simulink model "EV_thermal_charger_2015a_jmaab_Can02"  (R2015a)
settings: Solver=ode3  StartTime=0.0  StopTime=1800  FixedStep=sampling_time  RelTol=1e-3
PreLoadFcn:
  | %run('init_setting.m')
PostLoadFcn:
  | %set_param(gcs, 'SimulationCommand', 'update');
  | %load('save_param/save_P_Charger', 'P_Charger');
  | %load('save_param/save_T_User_set_temp_degC','T_User_set_temp_degC');
  | %load('save_param/save_ENV_PNT_PTTH_Temp_add_degC','ENV_PNT_PTTH_Temp_add_degC');
  | %load('save_param/save_ENV_PNT_CABIN_Temp_add_degC','ENV_PNT_CABIN_Temp_add_degC');
  | %load('save_param/save_ENV_PNT_PHI_Sunlight_W','ENV_PNT_PHI_Sunlight_W');
  | %load('save_param/save_ENV_PNT_Outside_Temp_ini_degC','ENV_PNT_Outside_Temp_ini_degC');
StartFcn:
  | tic
StopFcn:
  | toc
  | disp(['実時間の' num2str(toc/max(tout)) '倍'])
undefined symbols (not defined in the file or in its folder): BK_PNT_Pow_UL, BK_PNT_ReGene_vel_limit_DN_kmph, BK_PNT_ReGene_vel_limit_UP_kmph, BK_PNT_Tau_brake, Brk_LL, Brk_PGain, Brk_UL, BT_PNT_Hi_C_pol_hi_batt, BT_PNT_Hi_Capa_hi_batt_F, BT_PNT_Hi_ocv_SOC_hi_batt_OCV_V_table, BT_PNT_Hi_ocv_SOC_hi_batt_OCV_V_table_x_SOC, BT_PNT_Hi_R_hi_batt_cell, BT_PNT_Hi_R_pol_hi_batt, BT_PNT_Hi_SOC_MAX_hi_batt, BT_PNT_Hi_SOC_MIN_hi_batt, BT_PNT_Hi_SOC_START_hi_batt, BT_PNT_Lo_Capa_lo_batt_F, BT_PNT_Lo_ocv_SOC_lo_batt_OCV_V_table, BT_PNT_Lo_ocv_SOC_lo_batt_OCV_V_table_x_SOC, BT_PNT_Lo_R_lo_batt_ohm, BT_PNT_Lo_SOC_MAX_lo_batt, BT_PNT_Lo_SOC_MIN_lo_batt, BT_PNT_Lo_SOC_START_lo_batt, BTTH_CNT_P_BT_Heater_W, BTTH_CNT_P_BT_Heater_W_x_BTCells_degC, BTTH_CNT_Voltage_BTFan_V, BTTH_CNT_Voltage_BTFan_V_x_BTCells_degC, BTTH_PNT_BT_Heat_Resi_KpW, BTTH_PNT_BT_Heat_Resi_KpW_x_Wind_m3ps, BTTH_PNT_BT_Heater2BTCells_Heat_Resi_KpW, BTTH_PNT_BT_Heater_Heat_Capa_JpK, BTTH_PNT_BTBlock2BTAir_Heat_Resi_KpW, BTTH_PNT_BTBlock_Heat_Capa_JpK, BTTH_PNT_BTCells2BTBlock_Heat_Resi_KpW, BTTH_PNT_BTCells_Heat_Capa_JpK, BTTH_PNT_v_BTFan_Wind_vel_mps, BTTH_PNT_v_BTFan_Wind_vel_mps_x_V_BTFan, CATH_CNT_P_Aircon_W_LL, CATH_CNT_P_Aircon_W_UL, CATH_CNT_P_Gain_Aircon, CATH_CNT_P_Gain_PTC_Heater, CATH_CNT_P_Gain_SeatHT, CATH_CNT_P_PTC_Heater, CATH_CNT_P_PTC_Heater_W_LL, CATH_CNT_P_PTC_Heater_W_UL, CATH_CNT_P_PTC_Heater_x_T_Outside_temp_degC, CATH_CNT_P_SeatHT_W_LL, CATH_CNT_P_SeatHT_W_UL, CATH_CNT_PGain_Temp_blowout, CATH_CNT_T_Aircon_Indoor_degC, CATH_CNT_T_Aircon_Indoor_degC_x_T_blowout_degC, CATH_CNT_T_PTC_Heater_degC_UL, CATH_CNT_T_SeatHT_Temp_degC, CATH_CNT_T_SeatHT_Temp_degC_x_T_blowout_degC, CATH_CNT_V_HVAC_Fan, CATH_CNT_V_HVAC_Fan_x_T_blowout_degC, CATH_CNT_V_RDFan_V, CATH_CNT_V_RDFan_x_P_Aircon_W, CATH_PNT_Air_Convection_Heat_Resi_KpW, CATH_PNT_Air_Convection_Heat_Resi_x_mps ... (+141)
undefined symbols (not defined in the file): ACC_D_Gain, ACC_I_Gain, ACC_P_Gain
libraries: METI_Lib_vehicle_model x52, simulink x35
(part 2 of 6)

== system EV_thermal_charger_2015a_jmaab_Can02/Vehicle/EL_PNT ==
  note: 抵抗性負荷
  V_BT_Lo_PNT_V : Inport
  Add : Sum  Inputs=-+|
  Constant : Constant  Value=EL_PNT_R_bodyelec_lo
  Divide_0wari1 : Subsystem  mask(Divide_0割防止){}
      mask help:
      | 0割防止を行ったDivideブロックです。
      | 第2入力端子が0の場合、出力は0になります。
      mask Help:
      | 0割防止を行ったDivideブロックです。
      | 第2入力端子が0の場合、出力は0になります。
      mask Display:
      | port_label('input', 1, '×')
      | port_label('input', 2, '÷')
  Gain : Gain  Gain=-1
  Lo_body_elec_load_resi : Subsystem
  P_cal : METI_Lib_vehicle_model/P_cal  Type_energy=電気  Type_output_energy=損失  Power_name=Pl_  t_Workspace_Name=EL_PNT  P_VariableName=Pl_EL_PNT  Across_VariableName=V_EL_PNT  Throgh_VariableName=I_EL_PNT
  Terminator1 : Terminator
  V_Body_ground : Constant  Value=0
  I_EL_PNT_A : Outport
  wires:
  Divide_0wari1/1(Out1) -> Gain/1, P_cal/2
  V_BT_Lo_PNT_V/1 -> Add/2, P_cal/1
  Gain/1 -> I_EL_PNT_A/1  "I_EL_PNT_A"
  P_cal/1 -> Terminator1/1
  Constant/1 -> Divide_0wari1/2(In2)
  Add/1 -> Divide_0wari1/1(In1)
  V_Body_ground/1 -> Add/1

== system EV_thermal_charger_2015a_jmaab_Can02/Vehicle/INV_PT ==
  MG_CNT_out : Inport
  V_BT_Hi_PNT_V : Inport  Port=2
  T_INVTH_PNT_K : Inport  Port=3
  V_MG_PNT_AC_V : Inport  Port=4
  Bus Creator3 : BusCreator
  Bus Creator4 : BusCreator  Inputs=2
  Bus Selector8 : BusSelector  OutputSignals=tgt_I_MG_CNT_UPhase_A,tgt_k_MG_CNT_Vpradps,Power_factor_MG_CNT
  INV_PNT : Subsystem
  INV_sensor : Outport
  INV_MG : Outport  Port=2
  I_INV_PNT_AC_A : Outport  Port=3
  PHI_INV_PNT_W : Outport  Port=4
  I_INV_PNT_DC_A : Outport  Port=5
  wires:
  INV_PNT/2(Power_factor_INV_PNT) -> Bus Creator3/2, Bus Creator4/1  "Power_factor_INV_PNT"
  INV_PNT/3(V_INV_PNT_DC_V) -> Bus Creator3/3  "V_INV_PNT_DC_V"
  INV_PNT/1(k_INV_PNT_Vpradps) -> Bus Creator4/2, Bus Creator3/1  "k_INV_PNT_Vpradps"
  Bus Selector8/3 -> INV_PNT/3(Power_factor_MG_CNT)  "<Power_factor_MG_CNT>"
  T_INVTH_PNT_K/1 -> INV_PNT/5(T_INVTH_PNT_K)
  INV_PNT/4(I_INV_PNT_DC_A_1) -> Bus Creator3/4  "I_INV_PNT_DC_A_1"
  Bus Selector8/2 -> INV_PNT/2(tgt_k_MG_CNT_vpradps)  "<tgt_k_MG_CNT_Vpradps>"
  Bus Selector8/1 -> INV_PNT/1(tgt_I_MG_CNT_UPhase_A)  "<tgt_I_MG_CNT_UPhase_A>"
  V_BT_Hi_PNT_V/1 -> INV_PNT/4(V_BT_Hi_PNT_V)
  INV_PNT/5(I_INV_PNT_AC_A) -> I_INV_PNT_AC_A/1
  INV_PNT/7(I_INV_PNT_DC_A) -> I_INV_PNT_DC_A/1
  INV_PNT/6(PHI_INV_PNT_W) -> PHI_INV_PNT_W/1
  V_MG_PNT_AC_V/1 -> INV_PNT/6(V_MG_PNT_AC_V)
  Bus Creator3/1 -> INV_sensor/1  "INV_sensor"
  Bus Creator4/1 -> INV_MG/1  "INV_MG"
  MG_CNT_out/1 -> Bus Selector8/1

== system EV_thermal_charger_2015a_jmaab_Can02/Vehicle/MG_PNT ==
  INV_MG : Inport
  I_INV_PNT_AC_A : Inport  Port=2
  T_MGTH_PNT_K : Inport  Port=3
  w_TM_PNT_UP_radps : Inport  Port=4
  Bus Creator2 : BusCreator
  Bus Selector5 : BusSelector  OutputSignals=k_INV_PNT_Vpradps,Power_factor_INV_PNT
  MG_PNT : Subsystem
  MG_sensor : Outport
  Trq_MG_PNT_Nm : Outport  Port=2
  V_MG_PNT_AC_V : Outport  Port=3
  PHI_MG_PNT_W : Outport  Port=4
  wires:
  MG_PNT/3(V_MG_PNT_AC_V_1) -> Bus Creator2/3  "V_MG_PNT_AC_V_1"
  Bus Selector5/1 -> MG_PNT/1(k_MG_CNT_Vpradps)  "<k_INV_PNT_Vpradps>"
  T_MGTH_PNT_K/1 -> MG_PNT/4(T_MGTH_PNT_K)
  MG_PNT/1(w_MG_PNT_radps) -> Bus Creator2/1  "w_MG_PNT_radps"
  Bus Selector5/2 -> MG_PNT/2(Power_factor_INV_PNT)  "<Power_factor_INV_PNT>"
  MG_PNT/2("Trq_MG_PNT_Nm_1 ") -> Bus Creator2/2  "Trq_MG_PNT_Nm_1"
  MG_PNT/6("PHI_MG_PNT_W ") -> PHI_MG_PNT_W/1
  INV_MG/1 -> Bus Selector5/1
  MG_PNT/4(I_MG_PNT_AC_A) -> Bus Creator2/4  "I_MG_PNT_AC_A"
  Bus Creator2/1 -> MG_sensor/1  "MG_sensor"
  I_INV_PNT_AC_A/1 -> MG_PNT/3("I_INV_PNT_AC_A ")
  MG_PNT/5(Trq_MG_PNT_Nm) -> Trq_MG_PNT_Nm/1
  w_TM_PNT_UP_radps/1 -> MG_PNT/5(w_TM_PNT_UP_radps)
  MG_PNT/7("V_MG_PNT_AC_V ") -> V_MG_PNT_AC_V/1

== system EV_thermal_charger_2015a_jmaab_Can02/Vehicle/TR_PNT ==
  note: 車両を動かす側が正
  note: 車両を動かす側が正
  note: M (トルクNm) = F (力(N)） × r (タイヤ半径(m))
  note: omg (回転数rad/s) = v (車速m/s) / r (タイヤ半径(m))
  note: トルク⇔力変換
  note: 並進⇔回転変換
  note: 転がり抵抗
  "Trq_TR_PNT_Nm " : Inport
  Trq_TR_PNT_Nm 1 : Inport  Port=2
  v_VL_PNT_mps : Inport  Port=3
  Add5 : Sum
  Constant2 : Constant  Value=1/tire_r
  Product5 : Product  RndMeth=Zero
  Product6 : Product  RndMeth=Zero
  Sum2 : Sum  Inputs=-+|
  cal_roll_resi : METI_Lib_vehicle_model/vehicle_model/cal_roll_resi  Myu_tire=myu  Vehicle_Mass=M  Gravi_acc=g
  "F_TR_PNT_N " : Outport
  ｗ_TR_PNT_radps : Outport  Port=2
  tag scope: tScope_F_tire=global
  wires:
  "Trq_TR_PNT_Nm "/1 -> Add5/1
  Product5/1 -> ｗ_TR_PNT_radps/1  "w_TR_PNT_radps"
  v_VL_PNT_mps/1 -> Product5/1, cal_roll_resi/1
  Constant2/1 -> Product6/1, Product5/2
  Product6/1 -> Sum2/2
  cal_roll_resi/1 -> Sum2/1
  Sum2/1 -> "F_TR_PNT_N "/1, [tScope_F_tire]  "f_TR_PNT_N"
  Add5/1 -> Product6/2
  Trq_TR_PNT_Nm 1/1 -> Add5/2

== system EV_thermal_charger_2015a_jmaab_Can02/Vehicle/VL_PNT ==
  note: 空気抵抗
  note: 登坂抵抗
  note: 車両慣性
  F_TR_PNT_N : Inport
  Bus Creator : BusCreator  Inputs=1
  P_cal : METI_Lib_vehicle_model/P_cal  Type_energy=並進運動  Type_output_energy=出力  Power_name=Po_  t_Workspace_Name=VL_PNT_TIRE_MECK  P_VariableName=Po_VL_PNT_TIRE_MECK  Across_VariableName=v_VL_PNT_TIRE_MECK  Throgh_VariableName=F_VL_PNT_TIRE_MECK
  P_cal1 : METI_Lib_vehicle_model/P_cal  Type_energy=並進運動  Type_output_energy=損失  Power_name=Pl_  t_Workspace_Name=VL_PNT_AIR_RESI  P_VariableName=Pl_VL_PNT_AIR_RESI  Across_VariableName=v_VL_PNT_AIR_RESI  Throgh_VariableName=F_VL_PNT_AIR_RESI
  P_cal3 : METI_Lib_vehicle_model/P_cal  Type_energy=並進運動  Type_output_energy=損失  Power_name=Pl_  t_Workspace_Name=VL_PNT_GRAD_RESI_MECK  P_VariableName=Pl_VL_PNT_GRAD_RESI_MECK  Across_VariableName=v_VL_PNT_GRAD_RESI_MECK  Throgh_VariableName=F_VL_PNT_GRAD_RESI_MECK
  P_cal4 : METI_Lib_vehicle_model/P_cal  Type_energy=並進運動  Type_output_energy=出力  Power_name=Po_  t_Workspace_Name=VL_PNT_VL_MASS_MECK  P_VariableName=Po_VL_PNT_VL_MASS_MECK  Across_VariableName=v_VL_PNT_VL_MASS_MECK  Throgh_VariableName=F_VL_PNT_VL_MASS_MECK
  Sum1 : Sum  Inputs=-+|
  Sum3 : Sum  Inputs=-+|
  Terminator{2..5} (4 alike) : Terminator
  V_wind : Constant  Value=0
  angle : Constant  Value=0
  cal_Air_resi : METI_Lib_vehicle_model/vehicle_model/cal_Air_resi  Vel_max=200
  cal_Hill_Climbing_Resi : Subsystem
      mask Display: image(imread('picture\登坂.JPG'))
  cal_Vehicle_Mass : METI_Lib_vehicle_model/vehicle_model/cal_Vehicle_Mass  Vehicle_Mass=M
  mps2kmph : Gain  Gain=mps2kmph
  VL_PNT_sensor : Outport
  v_VL_PNT_mps : Outport  Port=2
  wires:
  P_cal4/1 -> Terminator2/1
  Sum1/1 -> cal_Vehicle_Mass/1, P_cal4/2
  P_cal1/1 -> Terminator5/1
  V_wind/1 -> cal_Air_resi/2
  cal_Air_resi/1 -> P_cal1/2, Sum3/1
  F_TR_PNT_N/1 -> P_cal/2, Sum3/2
  P_cal/1 -> Terminator3/1
  cal_Hill_Climbing_Resi/1(Out1) -> P_cal3/2, Sum1/1
  P_cal3/1 -> Terminator4/1
  Sum3/1 -> Sum1/2
  angle/1 -> cal_Hill_Climbing_Resi/1(In1)
  cal_Vehicle_Mass/1 -> mps2kmph/1, P_cal4/1, v_VL_PNT_mps/1, P_cal3/1, P_cal/1, P_cal1/1, cal_Air_resi/1  "v_VL_PNT_mps"
  mps2kmph/1 -> Bus Creator/1  "v_VL_PNT_kmph"
  Bus Creator/1 -> VL_PNT_sensor/1  "VL_PNT_sensor"

== system EV_thermal_charger_2015a_jmaab_Can02/Driver/Caliculate_Opeining_Accel/FB ==
  delta_v_VL_kmph : Inport
  Acc_D_Gain : Gain  Gain=D_Gain
  Acc_I_Gain : Gain  Gain=I_Gain
  Acc_P_Gain : Gain  Gain=P_Gain
  Acc_P_Gain1 : Gain  Gain=P_Gain
  Derivative : Derivative
  Filter : Subsystem  Commented=through
  Integrator : Integrator
  Memory : Memory
  Product1 : Product
  Saturation2 : Saturate  UpperLimit=1  LowerLimit=0
  Sum : Sum  Inputs=+++
  Terminator : Terminator
  FB_open_accel_per : Outport
  wires:
  Filter/1(Out1) -> Product1/2
  Saturation2/1 -> Acc_P_Gain/1
  Acc_P_Gain/1 -> Product1/1
  Sum/1 -> FB_open_accel_per/1
  Derivative/1 -> Acc_D_Gain/1
  Integrator/1 -> Acc_I_Gain/1
  delta_v_VL_kmph/1 -> Memory/1
  Acc_I_Gain/1 -> Sum/3
  Acc_D_Gain/1 -> Sum/2
  Acc_P_Gain1/1 -> Sum/1
  Memory/1 -> Saturation2/1, Filter/1(In1), Acc_P_Gain1/1, Integrator/1, Derivative/1
  Product1/1 -> Terminator/1

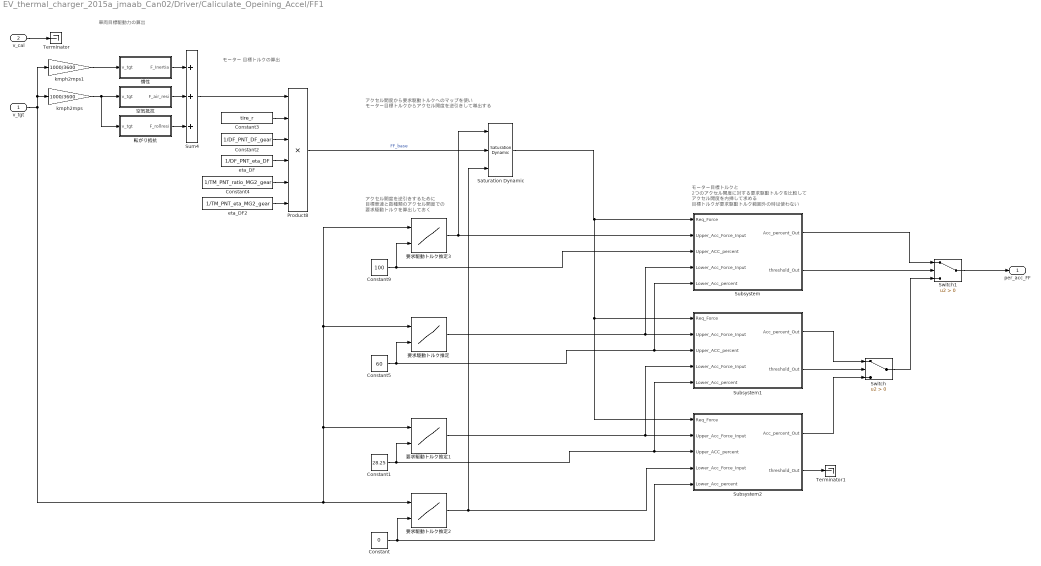
== system EV_thermal_charger_2015a_jmaab_Can02/Driver/Caliculate_Opeining_Accel/FF1 ==
  note: モーター目標トルクと
      | 2つのアクセル開度に対する要求駆動トルクを比較して
      | アクセル開度を内挿して求める
      | 目標トルクが要求駆動トルク範囲外の時は使わない
  note: アクセル開度を逆引きするために
      | 目標車速と数種類のアクセル開度での
      | 要求駆動トルクを算出しておく
  note: アクセル開度から要求駆動トルクへのマップを使い
      | モーター目標トルクからアクセル開度を逆引きして導出する
  note: モーター 目標トルクの算出
  note: 車両目標駆動力の算出
  v_tgt : Inport
  v_cal : Inport  Port=2
  Constant : Constant  Value=0
  Constant1 : Constant  Value=28.25
  Constant2 : Constant  Value=1/DF_PNT_DF_gear
  Constant3 : Constant  Value=tire_r
  Constant4 : Constant  Value=1/TM_PNT_ratio_MG2_gear
  Constant5 : Constant  Value=60
  Constant9 : Constant  Value=100
  Product8 : Product  Inputs=******  RndMeth=Zero
  Saturation Dynamic : simulink/Discontinuities/Saturation Dynamic  OutMin=[]  OutMax=[]  OutDataTypeStr=Inherit: Same as second input  OutDataType=fixdt(1, 16)  OutScaling=2^-10  DoSatur=off
  Subsystem : Subsystem
  Subsystem1 : Subsystem
  Subsystem2 : Subsystem
  Sum4 : Sum  Inputs=+++
  Switch : Switch  Criteria=u2 > Threshold
  Switch1 : Switch  Criteria=u2 > Threshold
  Terminator : Terminator
  Terminator1 : Terminator
  eta_DF : Constant  Value=1/DF_PNT_eta_DF
  eta_DF2 : Constant  Value=1/TM_PNT_eta_MG2_gear
  kmph2mps : Gain  Gain=1000/3600
  kmph2mps1 : Gain  Gain=1000/3600
  慣性 : Subsystem
  空気抵抗 : Subsystem
  要求駆動トルク推定{,1..3} (4 alike) : Lookup_n-D  BreakpointsForDimension1=VCU_CNT_trq_require_v_kmph  BreakpointsForDimension2=VCU_CNT_trq_require_accper  BeginIndexSearchUsingPreviousIndexResult=on  Table=VCU_CNT_trq_require_Nm  ExtrapMethod=Clip  InternalRulePriority=Speed  RndMeth=Simplest  InputSameDT=on
  転がり抵抗 : Subsystem
  per_acc_FF : Outport
  wires:
  v_cal/1 -> Terminator/1
  kmph2mps/1 -> 空気抵抗/1(v_tgt), 転がり抵抗/1(v_tgt)
  kmph2mps1/1 -> 慣性/1(v_tgt)
  慣性/1(F_Inertia) -> Sum4/1
  転がり抵抗/1(F_rollresi) -> Sum4/3
  空気抵抗/1(F_air_resi) -> Sum4/2
  Sum4/1 -> Product8/1
  v_tgt/1 -> kmph2mps/1, kmph2mps1/1, 要求駆動トルク推定2/1, 要求駆動トルク推定1/1, 要求駆動トルク推定3/1, 要求駆動トルク推定/1
  Constant/1 -> 要求駆動トルク推定2/2, Subsystem2/5(Lower_Acc_percent)
  Constant1/1 -> 要求駆動トルク推定1/2, Subsystem2/3(Upper_ACC_percent), Subsystem1/5(Lower_Acc_percent)
  Constant5/1 -> 要求駆動トルク推定/2, Subsystem1/3(Upper_ACC_percent), Subsystem/5(Lower_Acc_percent)
  要求駆動トルク推定1/1 -> Subsystem1/4(Lower_Acc_Force_Input), Subsystem2/2(Upper_Acc_Force_Input)
  要求駆動トルク推定2/1 -> Saturation Dynamic/3, Subsystem2/4(Lower_Acc_Force_Input)
  Product8/1 -> Saturation Dynamic/2  "FF_base"
  Saturation Dynamic/1 -> Subsystem1/1(Req_Force), Subsystem2/1(Req_Force), Subsystem/1(Req_Force)
  Constant9/1 -> 要求駆動トルク推定3/2, Subsystem/3(Upper_ACC_percent)
  要求駆動トルク推定/1 -> Subsystem1/2(Upper_Acc_Force_Input), Subsystem/4(Lower_Acc_Force_Input)
  要求駆動トルク推定3/1 -> Subsystem/2(Upper_Acc_Force_Input), Saturation Dynamic/1
  Switch/1 -> Switch1/3
  Switch1/1 -> per_acc_FF/1
  Subsystem/1(Acc_percent_Out) -> Switch1/1
  Subsystem/2(threshold_Out) -> Switch1/2
  Subsystem1/2(threshold_Out) -> Switch/2
  Subsystem1/1(Acc_percent_Out) -> Switch/1
  Subsystem2/1(Acc_percent_Out) -> Switch/3
  Subsystem2/2(threshold_Out) -> Terminator1/1
  Constant3/1 -> Product8/2
  Constant2/1 -> Product8/3
  eta_DF/1 -> Product8/4
  Constant4/1 -> Product8/5
  eta_DF2/1 -> Product8/6

== system EV_thermal_charger_2015a_jmaab_Can02/Driver/Caliculate_Opeining_Accel/stopmode_calc ==
  note: 停車時（＝目標車速が閾値以下の時）は
      | アクセルを踏まないようにする
  FF_FB_acc_per : Inport
  target_v_VL_kmph : Inport  Port=2
  Compare To Zero : simulink/Logic and Bit Operations/Compare To Zero  relop=>  OutDataTypeStr=boolean
  Constant2 : Constant  Value=0
  Constant6 : Constant  Value=Driver_Brake_Switch_Const2
  Subtract : Sum  Inputs=+-
  Switch : Switch  Criteria=u2 > Threshold
  open_accel_per : Outport
  wires:
  Subtract/1 -> Compare To Zero/1
  Switch/1 -> open_accel_per/1
  Compare To Zero/1 -> Switch/2
  Constant2/1 -> Switch/3
  Constant6/1 -> Subtract/2
  target_v_VL_kmph/1 -> Subtract/1
  FF_FB_acc_per/1 -> Switch/1

== system EV_thermal_charger_2015a_jmaab_Can02/Vehicle/ATM_PNT/degC->K ==
  degC : Inport
  Constant2 : Constant  Value=degC2K
  Sum : Sum  Inputs=++|
  K : Outport
  wires:
  degC/1 -> Sum/2
  Constant2/1 -> Sum/1
  Sum/1 -> K/1

== system EV_thermal_charger_2015a_jmaab_Can02/Vehicle/BAT_Hi_PNT/BT_Hi_PNT ==
  note: SOC算出
  note: 内部抵抗
  note: OCV電圧算出
  I_BT_Hi_PNT_A : Inport
  T_BC_PNT_K : Inport  Port=2
  Cal_SOC : Subsystem
  Capa_batt(Ah) : Constant  Value=BT_PNT_Hi_Capa_hi_batt_F
  Gain : Gain  Gain=-1
  Memory6 : Memory  InheritSampleTime=on
  P_cal : METI_Lib_vehicle_model/P_cal  Type_energy=電気  Type_output_energy=出力  Power_name=Po_  t_Workspace_Name=BT_HI_PNT_ELEC  P_VariableName=Po_BT_HI_PNT_ELEC  Across_VariableName=V_BT_HI_PNT_ELEC  Throgh_VariableName=I_BT_HI_PNT_ELEC
  P_cal1 : METI_Lib_vehicle_model/P_cal  Type_energy=電気  Type_output_energy=損失  Power_name=Pl_  t_Workspace_Name=BT_PNT_HI_ELEC_LOSS  P_VariableName=Pl_BT_PNT_HI_ELEC_LOSS  Across_VariableName=V_BT_PNT_HI_ELEC_LOSS  Throgh_VariableName=I_BT_PNT_HI_ELEC_LOSS
  Product : Product
  SOC_MAX(%) : Constant  Value=BT_PNT_Hi_SOC_MAX_hi_batt
  SOC_MIN(%) : Constant  Value=BT_PNT_Hi_SOC_MIN_hi_batt
  SOC_START(%) : Constant  Value=BT_PNT_Hi_SOC_START_hi_batt
  Signal Specification : SignalSpecification
  Subsystem : Subsystem
  Sum : Sum
  Terminator1 : Terminator
  Terminator2 : Terminator
  map_OCV : Lookup  InputValues=BT_PNT_Hi_ocv_SOC_hi_batt_OCV_V_table_x_SOC  Table=BT_PNT_Hi_ocv_SOC_hi_batt_OCV_V_table  LookUpMeth=Interpolation-Use End Values
  V_BT_Hi_PNT_V_1 : Outport
  SOC_BT_Hi_PNT_per : Outport  Port=2
  V_BT_Hi_PNT_V : Outport  Port=3
  PHI_BT_Hi_PNT_W : Outport  Port=4
  tag scope: tScope_I_BT_HI_PNT_A=global, tScope_PHI_BT_HI_PNT_W=global, tScope_P_BT_HI_PNT_W=global, tScope_SOC_HiBatt=global, tScope_V_BT_HI_PNT_V=global
  wires:
  Capa_batt(Ah)/1 -> Cal_SOC/2(Capa_batt)
  SOC_START(%)/1 -> Cal_SOC/3(SOC_st)
  SOC_MAX(%)/1 -> Cal_SOC/4(SOC_MAX)
  SOC_MIN(%)/1 -> Cal_SOC/5(SOC_MIN)
  Sum/1 -> V_BT_Hi_PNT_V_1/1, Product/1, Signal Specification/1, [tScope_V_BT_HI_PNT_V], P_cal/1  "volt_BT_HI_PNT_V"
  map_OCV/1 -> Sum/1
  Subsystem/1(V_BT_PNT_V) -> P_cal1/1, Sum/2
  P_cal/1 -> Terminator2/1
  P_cal1/1 -> PHI_BT_Hi_PNT_W/1, [tScope_PHI_BT_HI_PNT_W]  "PHI_BT_Hi_PNT_W"
  I_BT_Hi_PNT_A/1 -> Gain/1, Memory6/1
  Cal_SOC/1(SOC_out) -> SOC_BT_Hi_PNT_per/1, [tScope_SOC_HiBatt], map_OCV/1  "SOC_BT_HI_PNT_PCT"
  Memory6/1 -> Subsystem/1(I_BT_PNT_A), P_cal1/2, Cal_SOC/1(I_BT_PNT_A)
  T_BC_PNT_K/1 -> Terminator1/1
  Product/1 -> [tScope_P_BT_HI_PNT_W]
  Gain/1 -> [tScope_I_BT_HI_PNT_A], P_cal/2, Product/2
  Signal Specification/1 -> V_BT_Hi_PNT_V/1  "V_BT_Hi_PNT_V"

== system EV_thermal_charger_2015a_jmaab_Can02/Vehicle/BTTH/BTTH_PNT ==
  tgt_P_BTTH_CNT_BTHeater_W : Inport
  V_BTTH_CNT_BTFan_V : Inport  Port=2
  V_BT_Lo_PNT_V : Inport  Port=3
  PHI_BT_HI_PNT_W : Inport  Port=4
  T_ATM_PNT_BB_K : Inport  Port=5
  T_ATM_PNT_BF_K : Inport  Port=6
  <ini_T_Environment_Outside_degC> : Inport  Port=7
  BB_PNT : Subsystem
  BC_PNT : Subsystem
  BF_PNT : Subsystem
  BH_PNT : Subsystem
  K->degC : Subsystem
  K->degC1 : Subsystem
  I_BTTH_PNT_A : Outport
  PHI_BB_PNT_ATM_W : Outport  Port=2
  PHI_BF_PNT_ATM_W : Outport  Port=3
  T_BC_PNT_degC : Outport  Port=4
  T_BC_PNT_K : Outport  Port=5
  tag scope: tScope_PHI_BTTH_PNT_BT2AIR_W=global, tScope_T_BTBlock_degC=global, tScope_T_BTCells_degC=global
  wires:
  K->degC/1(degC) -> [tScope_T_BTCells_degC], T_BC_PNT_degC/1  "T_BTCells_degC"
  K->degC1/1(degC) -> [tScope_T_BTBlock_degC]
  <ini_T_Environment_Outside_degC>/1 -> BH_PNT/1(ini_T_Environment_Outside_degC), BC_PNT/3(ini_T_Environment_Outside_degC), BB_PNT/1(ini_T_Environment_Outside_degC)
  tgt_P_BTTH_CNT_BTHeater_W/1 -> BH_PNT/2(tgt_P_BTTH_CNT_BTHeater_W)  "tgt_P_BTTH_CNT_BTHeater_W"
  V_BT_Lo_PNT_V/1 -> BH_PNT/3(V_BT_Lo_PNT_V)
  BH_PNT/2(I_BTTH_PNT_A) -> I_BTTH_PNT_A/1
  PHI_BT_HI_PNT_W/1 -> BC_PNT/5(PHI_BT_HI_PNT_W)
  BH_PNT/1(PHI_BTCells_Resi1_W) -> BC_PNT/4(PHI_BTCells2_W)
  BC_PNT/3(T_BC_PNT_K) -> T_BC_PNT_K/1
  BC_PNT/5(T_BTCells2_K) -> BH_PNT/4(T_BTCells_Resi1_K)
  BC_PNT/4(T_BTCCell_K) -> K->degC/1(K)
  V_BTTH_CNT_BTFan_V/1 -> BF_PNT/1(V_BTTH_CNT_BTFan_V)  "V_BTTH_CNT_BTFan_V"
  BC_PNT/1(T_BTCells4_K) -> BF_PNT/3(T_BT_Fan_Resi2_K)
  T_ATM_PNT_BF_K/1 -> BF_PNT/2(T_ATM_PNT_BF_K)
  BF_PNT/1(PHI_BT_Fan_Resi2_W) -> BC_PNT/1(PHI_BTCells4_W)
  BF_PNT/2(PHI_BF_PNT_ATM_W) -> PHI_BF_PNT_ATM_W/1
  BB_PNT/2(PHI_BB_PNT_ATM_W) -> PHI_BB_PNT_ATM_W/1, [tScope_PHI_BTTH_PNT_BT2AIR_W]
  BC_PNT/2(PHI_BTBlock_Resi1_W) -> BB_PNT/3(PHI_BTBlock1_W)
  T_ATM_PNT_BB_K/1 -> BB_PNT/2(T_ATM_PNT_BB_K)
  BB_PNT/1(T_BTBlock1_K) -> BC_PNT/2(T_BTBlock_Resi1_K)
  BB_PNT/3(T_BTBlock2_K) -> K->degC1/1(K)

== system EV_thermal_charger_2015a_jmaab_Can02/Vehicle/BT_Lo_PNT/BT_Lo_PNT ==
  note: SOC算出
  note: 内部抵抗
  note: OCV電圧算出
  I_BT_Lo_PNT_A : Inport
  Cal_SOC : Subsystem
  Capa_batt(Ah) : Constant  Value=BT_PNT_Lo_Capa_lo_batt_F
  Memory6 : Memory  InheritSampleTime=on
  P_cal : METI_Lib_vehicle_model/P_cal  Type_energy=電気  Type_output_energy=出力  Power_name=Po_  t_Workspace_Name=BT_PNT_Lo_ELEC  P_VariableName=Po_BT_PNT_Lo_ELEC  Across_VariableName=V_BT_PNT_Lo_ELEC  Throgh_VariableName=I_BT_PNT_Lo_ELEC
  P_cal1 : METI_Lib_vehicle_model/P_cal  Type_energy=電気  Type_output_energy=損失  Power_name=Pl_  t_Workspace_Name=BT_PNT_Lo_ELEC_LOSS  P_VariableName=Pl_BT_PNT_Lo_ELEC_LOSS  Across_VariableName=V_BT_PNT_Lo_ELEC_LOSS  Throgh_VariableName=I_BT_PNT_Lo_ELEC_LOSS
  SOC_MAX(%) : Constant  Value=BT_PNT_Lo_SOC_MAX_lo_batt
  SOC_MIN(%) : Constant  Value=BT_PNT_Lo_SOC_MIN_lo_batt
  SOC_START(%) : Constant  Value=BT_PNT_Lo_SOC_START_lo_batt
  Signal Specification : SignalSpecification
  Subsystem : Subsystem
  Sum : Sum
  Terminator1 : Terminator
  Terminator2 : Terminator
  map_OCV : Lookup  InputValues=BT_PNT_Lo_ocv_SOC_lo_batt_OCV_V_table_x_SOC  Table=BT_PNT_Lo_ocv_SOC_lo_batt_OCV_V_table  LookUpMeth=Interpolation-Use End Values
  "V_BT_Lo_PNT_V " : Outport
  tag scope: tScope_SOC_LoBatt=global
  wires:
  Capa_batt(Ah)/1 -> Cal_SOC/2(Capa_batt)
  SOC_START(%)/1 -> Cal_SOC/3(SOC_st)
  SOC_MAX(%)/1 -> Cal_SOC/4(SOC_MAX)
  SOC_MIN(%)/1 -> Cal_SOC/5(SOC_MIN)
  Sum/1 -> P_cal/1, Signal Specification/1  "volt_BT_PNT_Lo_V"
  map_OCV/1 -> Sum/1
  Subsystem/1(V_BT_PNT_Lo_V) -> P_cal1/1, Sum/2
  P_cal/1 -> Terminator2/1
  P_cal1/1 -> Terminator1/1
  I_BT_Lo_PNT_A/1 -> Memory6/1, P_cal/2
  Cal_SOC/1(SOC_out) -> map_OCV/1, [tScope_SOC_LoBatt]  "SOC_BT_PNT_Lo_PCT"
  Memory6/1 -> Subsystem/1(I_BT_PNT_Lo_A), P_cal1/2, Cal_SOC/1(I_Lo_BT_PNT_A)
  Signal Specification/1 -> "V_BT_Lo_PNT_V "/1  "V_BT_Lo_PNT_V"

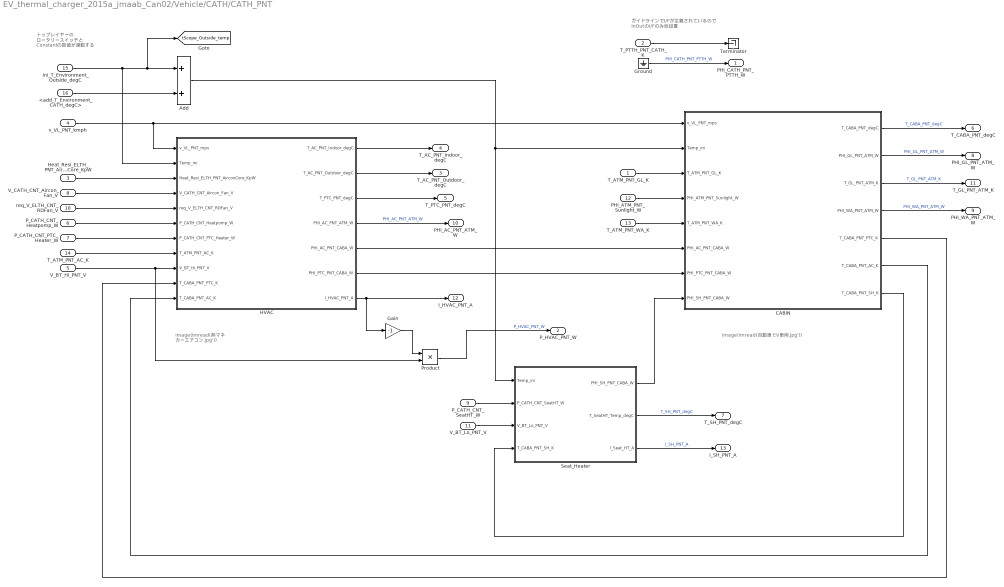
== system EV_thermal_charger_2015a_jmaab_Can02/Vehicle/CATH/CATH_PNT ==
  note: image(imread('自動車 EV車両.jpg'))
  note: image(imread('熱マネ カーエアコン.jpg'))
  note: トップレイヤーの
      | ロータリースイッチと
      | Constantの数値が連動する
  note: ガイドラインでI/Fが定義されているので
      | InOutのI/Fのみ仮設置
  T_ATM_PNT_GL_K : Inport
  T_PTTH_PNT_CATH_K : Inport  Port=2
  Heat_Resi_ELTH_PNT_AirconCore_KpW : Inport  Port=3
  v_VL_PNT_kmph : Inport  Port=4
  V_BT_Hi_PNT_V : Inport  Port=5
  P_CATH_CNT_Heatpomp_W : Inport  Port=6
  P_CATH_CNT_PTC_Heater_W : Inport  Port=7
  V_CATH_CNT_Aircon_Fan_V : Inport  Port=8
  P_CATH_CNT_SeatHT_W : Inport  Port=9
  req_V_ELTH_CNT_RDFan_V : Inport  Port=10
  V_BT_Lo_PNT_V : Inport  Port=11
  PHI_ATM_PNT_Sunlight_W : Inport  Port=12
  T_ATM_PNT_WA_K : Inport  Port=13
  T_ATM_PNT_AC_K : Inport  Port=14
  ini_T_Environment_Outside_degC : Inport  Port=15
  <add_T_Environment_CATH_degC> : Inport  Port=16
  Add : Sum
  CABIN : Subsystem
  Gain : Gain  Gain=-1
  Ground : Ground
  HVAC : Subsystem
  Product : Product
  Seat_Heater : Subsystem
  Terminator : Terminator
  PHI_CATH_PNT_PTTH_W : Outport
  P_HVAC_PNT_W : Outport  Port=2
  T_AC_PNT_Outdoor_degC : Outport  Port=3
  T_AC_PNT_Indoor_degC : Outport  Port=4
  T_PTC_PNT_degC : Outport  Port=5
  T_CABA_PNT_degC : Outport  Port=6
  T_SH_PNT_degC : Outport  Port=7
  PHI_GL_PNT_ATM_W : Outport  Port=8
  PHI_WA_PNT_ATM_W : Outport  Port=9
  PHI_AC_PNT_ATM_W : Outport  Port=10
  T_GL_PNT_ATM_K : Outport  Port=11
  I_HVAC_PNT_A : Outport  Port=12
  I_SH_PNT_A : Outport  Port=13
  tag scope: tScope_Outside_temp=global
  wires:
  HVAC/7(I_HVAC_PNT_A) -> I_HVAC_PNT_A/1, Gain/1
  Product/1 -> P_HVAC_PNT_W/1  "P_HVAC_PNT_W"
  CABIN/6(T_CABA_PNT_AC_K) -> HVAC/11(T_CABA_PNT_AC_K)
  CABIN/5(T_CABA_PNT_PTC_K) -> HVAC/10(T_CABA_PNT_PTC_K)
  V_BT_Lo_PNT_V/1 -> Seat_Heater/3(V_BT_Lo_PNT_V)
  Seat_Heater/3(I_Seat_HT_A) -> I_SH_PNT_A/1  "I_SH_PNT_A"
  P_CATH_CNT_SeatHT_W/1 -> Seat_Heater/2(P_CATH_CNT_SeatHT_W)
  CABIN/7(T_CABA_PNT_SH_K) -> Seat_Heater/4(T_CABA_PNT_SH_K)
  T_ATM_PNT_AC_K/1 -> HVAC/8(T_ATM_PNT_AC_K)
  CABIN/1(T_CABA_PNT_degC) -> T_CABA_PNT_degC/1  "T_CABA_PNT_degC"
  CABIN/3(T_GL_PNT_ATM_K) -> T_GL_PNT_ATM_K/1  "T_GL_PNT_ATM_K"
  PHI_ATM_PNT_Sunlight_W/1 -> CABIN/4(PHI_ATM_PNT_Sunlight_W)
  T_ATM_PNT_GL_K/1 -> CABIN/3(T_ATM_PNT_GL_K)
  CABIN/2(PHI_GL_PNT_ATM_W) -> PHI_GL_PNT_ATM_W/1  "PHI_GL_PNT_ATM_W"
  T_ATM_PNT_WA_K/1 -> CABIN/5(T_ATM_PNT_WA_K)
  CABIN/4(PHI_WA_PNT_ATM_W) -> PHI_WA_PNT_ATM_W/1  "PHI_WA_PNT_ATM_W"
  Seat_Heater/1(PHI_SH_PNT_CABA_W) -> CABIN/8(PHI_SH_PNT_CABA_W)
  HVAC/6(PHI_PTC_PNT_CABA_W) -> CABIN/7(PHI_PTC_PNT_CABA_W)
  HVAC/5(PHI_AC_PNT_CABA_W) -> CABIN/6(PHI_AC_PNT_CABA_W)
  HVAC/4(PHI_AC_PNT_ATM_W) -> PHI_AC_PNT_ATM_W/1  "PHI_AC_PNT_ATM_W"
  v_VL_PNT_kmph/1 -> HVAC/1(v_VL_PNT_mps), CABIN/1(v_VL_PNT_mps)
  V_CATH_CNT_Aircon_Fan_V/1 -> HVAC/4(V_CATH_CNT_Aircon_Fan_V)
  req_V_ELTH_CNT_RDFan_V/1 -> HVAC/5(req_V_ELTH_CNT_RDFan_V)
  P_CATH_CNT_Heatpomp_W/1 -> HVAC/6(P_CATH_CNT_Heatpomp_W)
  P_CATH_CNT_PTC_Heater_W/1 -> HVAC/7(P_CATH_CNT_PTC_Heater_W)
  HVAC/1(T_AC_PNT_Indoor_degC) -> T_AC_PNT_Indoor_degC/1
  HVAC/2(T_AC_PNT_Outdoor_degC) -> T_AC_PNT_Outdoor_degC/1
  HVAC/3(T_PTC_PNT_degC) -> T_PTC_PNT_degC/1
  V_BT_Hi_PNT_V/1 -> HVAC/9(V_BT_Hi_PNT_V), Product/2
  Seat_Heater/2(T_SeatHT_Temp_degC) -> T_SH_PNT_degC/1  "T_SH_PNT_degC"
  Heat_Resi_ELTH_PNT_AirconCore_KpW/1 -> HVAC/3(Heat_Resi_ELTH_PNT_AirconCore_KpW)
  Ground/1 -> PHI_CATH_PNT_PTTH_W/1  "PHI_CATH_PNT_PTTH_W"
  T_PTTH_PNT_CATH_K/1 -> Terminator/1
  ini_T_Environment_Outside_degC/1 -> HVAC/2(Temp_ini), Add/1, [tScope_Outside_temp]
  <add_T_Environment_CATH_degC>/1 -> Add/2
  Add/1 -> Seat_Heater/1(Temp_ini), CABIN/2(Temp_ini)
  Gain/1 -> Product/1

== system EV_thermal_charger_2015a_jmaab_Can02/Vehicle/CNT/BK_CNT ==
  DriverDmnd : Inport
  BK_CNT : Subsystem
  Bus Creator11 : BusCreator  Inputs=1
  Bus Selector14 : BusSelector  OutputSignals=open_brake_Driver_per
  Bus Selector4 : BusSelector  OutputSignals=F_VCU_CNT_re_break_N
  BK_CNT_out : Outport
  wires:
  Bus Selector4/1 -> BK_CNT/2(F_VCU_CNT_re_brake_N)  "<F_VCU_CNT_re_break_N>"
  Bus Selector14/1 -> BK_CNT/1(open_brake_Driver_per)  "<open_brake_Driver_per>"
  DriverDmnd/1 -> Bus Selector14/1
  BK_CNT/1(open_brake_BK_CNT_per) -> Bus Creator11/1  "open_brake_BK_CNT_per"
  Bus Creator11/1 -> BK_CNT_out/1  "BK_CNT_out"
  [BK_CNT_CAN_Rx] -> Bus Selector4/1

== system EV_thermal_charger_2015a_jmaab_Can02/Vehicle/CNT/BTTH_CNT ==
  BTTH_sensor : Inport
  BTTH_CNT : Subsystem
  Bus Creator1 : BusCreator  Inputs=2
  Bus Selector2 : BusSelector  OutputSignals=T_BC_PNT_degC
  BTTH_CNT_out : Outport
  wires:
  BTTH_CNT/2(V_BTTH_CNT_BTFan_V) -> Bus Creator1/2  "V_BTTH_CNT_BTFan_V"
  Bus Selector2/1 -> BTTH_CNT/1(T_BC_PNT_degC)  "<T_BC_PNT_degC>"
  BTTH_CNT/1(tgt_P_BTTH_CNT_BTHeater_W) -> Bus Creator1/1  "tgt_P_BTTH_CNT_BTHeater_W"
  Bus Creator1/1 -> BTTH_CNT_out/1  "BTTH_CNT_out"
  BTTH_sensor/1 -> Bus Selector2/1

== system EV_thermal_charger_2015a_jmaab_Can02/Vehicle/CNT/CAN ==
  BK_CNT : Subsystem
  CATH_CNT : Subsystem
  ELTH_CNT : Subsystem
  MG_CNT : Subsystem
  PwtrCAN : Subsystem
  "VCU_CNT " : Subsystem
  VehCAN : Subsystem
  wires:
  "VCU_CNT "/1(VCU_CNT_CAN_Tx) -> PwtrCAN/1(VCU_CNT_CAN_Tx)
  CATH_CNT/1(CATH_CNT_CAN_Tx) -> VehCAN/1(CATH_CNT_CAN_Tx)
  PwtrCAN/1(PwtrCAN) -> MG_CNT/1(PwtrCAN), BK_CNT/1(PwtrCAN)
  VehCAN/1(VenCAN) -> ELTH_CNT/1(VenCAN)

== system EV_thermal_charger_2015a_jmaab_Can02/Vehicle/CNT/CATH_CNT ==
  CATH_sensor : Inport
  ATM_PNT_sensor : Inport  Port=2
  VL_sensor : Inport  Port=3
  Driver_Input : Inport  Port=4
  Bus Creator : BusCreator  Inputs=1
  Bus Creator5 : BusCreator  Inputs=5
  Bus Selector1 : BusSelector  OutputSignals=T_ATM_PNT_Outside_degC
  Bus Selector16 : BusSelector  OutputSignals=v_VL_PNT_kmph
  Bus Selector3 : BusSelector  OutputSignals=T_CABA_PNT_degC,T_SH_PNT_degC,T_AC_PNT_Indoor_degC,T_PTC_PNT_degC
  Bus Selector5 : BusSelector  OutputSignals=tSetting_P_Charger,tSetting_T_User_set_temp_degC
  CATH_CNT : Subsystem
  CATH_CNT_out : Outport
  tag scope: CATH_CNT_CAN_Tx=scoped
  wires:
  Bus Creator5/1 -> CATH_CNT_out/1  "CATH_CNT_out"
  VL_sensor/1 -> Bus Selector16/1
  Bus Selector5/1 -> CATH_CNT/1(tSetting_P_Charger)  "<tSetting_P_Charger>"
  CATH_CNT/3(req_V_CATH_CNT_RDFan_V) -> Bus Creator/1, Bus Creator5/3  "req_V_CATH_CNT_RDFan_V"
  Bus Selector3/4 -> CATH_CNT/7(T_PTC_PNT_degC)  "<T_PTC_PNT_degC>"
  CATH_CNT/1(V_CATH_CNT_Aircon_Fan_V) -> Bus Creator5/1  "V_CATH_CNT_Aircon_Fan_V"
  CATH_CNT/4(P_CATH_CNT_PTC_Heater_W) -> Bus Creator5/4  "P_CATH_CNT_PTC_Heater_W"
  CATH_CNT/2(P_CATH_CNT_Heatpomp_W) -> Bus Creator5/2  "P_CATH_CNT_Heatpomp_W"
  Bus Selector5/2 -> CATH_CNT/2(tSetting_T_User_set_temp_degC)  "<tSetting_T_User_set_temp_degC>"
  Bus Selector16/1 -> CATH_CNT/8(v_VL_PNT_kmph)  "<v_VL_PNT_kmph>"
  Bus Selector3/1 -> CATH_CNT/4(T_CABA_PNT_degC)  "<T_CABA_PNT_degC>"
  Bus Selector3/2 -> CATH_CNT/5(T_SH_PNT_degC)  "<T_SH_PNT_degC>"
  Bus Selector3/3 -> CATH_CNT/6(T_AC_PNT_Indoor_degC)  "<T_AC_PNT_Indoor_degC>"
  CATH_CNT/5(P_CATH_CNT_SeatHT_W) -> Bus Creator5/5  "P_CATH_CNT_SeatHT_W"
  Driver_Input/1 -> Bus Selector5/1
  Bus Creator/1 -> [CATH_CNT_CAN_Tx]  "CATH_CNT_CAN_Tx"
  CATH_sensor/1 -> Bus Selector3/1
  ATM_PNT_sensor/1 -> Bus Selector1/1
  Bus Selector1/1 -> CATH_CNT/3(T_ATM_PNT_Outside_degC)  "<T_ATM_PNT_Outside_degC>"

== system EV_thermal_charger_2015a_jmaab_Can02/Vehicle/CNT/CHG_CNT ==
  DriverDmnd : Inport
  CHG_PNT_sensor : Inport  Port=2
  BT_Hi_PNT_sensor : Inport  Port=3
  Bus Creator22 : BusCreator  Inputs=1
  Bus Selector1 : BusSelector  OutputSignals=tSetting_P_Charger
  Bus Selector2 : BusSelector  OutputSignals=V_CHG_PNT_V
  Bus Selector3 : BusSelector  OutputSignals=SOC_BT_Hi_PNT_per
  CHG_CNT : Subsystem
  CHG_CNT_out : Outport
  wires:
  Bus Creator22/1 -> CHG_CNT_out/1  "CHG_CNT_out"
  CHG_CNT/1(tgt_I_CHG_CNT_Charge_A) -> Bus Creator22/1  "tgt_I_CHG_CNT_Charge_A"
  Bus Selector1/1 -> CHG_CNT/1(tSetting_P_Charger)  "<tSetting_P_Charger>"
  DriverDmnd/1 -> Bus Selector1/1
  BT_Hi_PNT_sensor/1 -> Bus Selector3/1
  CHG_PNT_sensor/1 -> Bus Selector2/1
  Bus Selector2/1 -> CHG_CNT/2(V_CHG_PNT_V)  "<V_CHG_PNT_V>"
  Bus Selector3/1 -> CHG_CNT/3(SOC_BT_Hi_PNT_per)  "<SOC_BT_Hi_PNT_per>"

== system EV_thermal_charger_2015a_jmaab_Can02/Vehicle/CNT/ELTH_CNT ==
  PTTH_sensor : Inport
  Bus Creator12 : BusCreator  Inputs=2
  Bus Selector10 : BusSelector  OutputSignals=req_V_CATH_CNT_RDFan_V
  Bus Selector13 : BusSelector  OutputSignals=T_RDTH_PNT_RDCoolant_degC
  ELTH_CNT : Subsystem
  ELTH_CNT_out : Outport
  wires:
  ELTH_CNT/1(req_V_ELTH_CNT_RDFan_V) -> Bus Creator12/1  "req_V_ELTH_CNT_RDFan_V"
  ELTH_CNT/2(V_ELTH_CNT_WP_V) -> Bus Creator12/2  "V_ELTH_CNT_WP_V"
  Bus Selector10/1 -> ELTH_CNT/2(req_V_CATH_CNT_RDFan_V)  "<req_V_CATH_CNT_RDFan_V>"
  Bus Selector13/1 -> ELTH_CNT/1(T_RDTH_PNT_RDCoolant_degC)  "<T_RDTH_PNT_RDCoolant_degC>"
  Bus Creator12/1 -> ELTH_CNT_out/1  "ELTH_CNT_out"
  [ELTH_CNT_CAN_Rx] -> Bus Selector10/1
  PTTH_sensor/1 -> Bus Selector13/1

== system EV_thermal_charger_2015a_jmaab_Can02/Vehicle/CNT/MG_CNT ==
  MG_sensor : Inport
  INV_sensor : Inport  Port=2
  Bus Creator6 : BusCreator  Inputs=3
  Bus Selector1 : BusSelector  OutputSignals=tgt_Trq_VCU_CNT_MG_Nm
  Bus Selector2 : BusSelector  OutputSignals=w_MG_PNT_radps
  Bus Selector3 : BusSelector  OutputSignals=V_INV_PNT_DC_V
  MG_CNT : Subsystem
  MG_CNT_out : Outport
  wires:
  Bus Selector1/1 -> MG_CNT/1(tgt_Trq_VCU_CNT_MG_Nm)  "<tgt_Trq_VCU_CNT_MG_Nm>"
  MG_CNT/2(tgt_k_MG_CNT_Vpradps) -> Bus Creator6/2  "tgt_k_MG_CNT_Vpradps"
  MG_CNT/3(tgt_I_MG_CNT_UPhase_A) -> Bus Creator6/3  "tgt_I_MG_CNT_UPhase_A"
  MG_CNT/1(Power_factor_MG_CNT) -> Bus Creator6/1  "Power_factor_MG_CNT"
  Bus Creator6/1 -> MG_CNT_out/1  "MG_CNT_out"
  MG_sensor/1 -> Bus Selector2/1
  INV_sensor/1 -> Bus Selector3/1
  Bus Selector2/1 -> MG_CNT/2(w_MG_PNT_radps)  "<w_MG_PNT_radps>"
  Bus Selector3/1 -> MG_CNT/3(V_INV_PNT_DC_V)  "<V_INV_PNT_DC_V>"
  [MG_CNT_CAN_Rx] -> Bus Selector1/1

== system EV_thermal_charger_2015a_jmaab_Can02/Vehicle/CNT/VCU_CNT ==
  Driver_Input : Inport
  VL_sensor : Inport  Port=2
  DCDC_PNT_sensor : Inport  Port=3
  MG_sensor : Inport  Port=4
  CATH_sensor : Inport  Port=5
  BT_Hi_PNT_sensor : Inport  Port=6
  Bus Creator : BusCreator  Inputs=2
  Bus Selector1 : BusSelector  OutputSignals=w_MG_PNT_radps
  Bus Selector11 : BusSelector  OutputSignals=v_VL_PNT_kmph
  Bus Selector12 : BusSelector  OutputSignals=open_brake_Driver_per,open_accel_Driver_per
  Bus Selector2 : BusSelector  OutputSignals=SOC_BT_Hi_PNT_per
  Bus Selector3 : BusSelector  OutputSignals=P_DCDC_PNT_W
  Bus Selector4 : BusSelector  OutputSignals=P_HVAC_PNT_W
  VCU_CNT : Subsystem
  tag scope: VCU_CNT_CAN_Tx=scoped
  wires:
  Bus Selector12/2 -> VCU_CNT/2(open_accel_Driver_per)  "<open_accel_Driver_per>"
  Bus Selector12/1 -> VCU_CNT/1(open_break_Driver_per)  "<open_brake_Driver_per>"
  VCU_CNT/1(F_VCU_CNT_re_break_N) -> Bus Creator/1  "F_VCU_CNT_re_break_N"
  Driver_Input/1 -> Bus Selector12/1
  VCU_CNT/2(tgt_Trq_VCU_CNT_MG_Nm) -> Bus Creator/2  "tgt_Trq_VCU_CNT_MG_Nm"
  Bus Selector11/1 -> VCU_CNT/3(v_VL_PNT_kmph)  "<v_VL_PNT_kmph>"
  Bus Creator/1 -> [VCU_CNT_CAN_Tx]  "VCU_CNT_CAN_Tx"
  VL_sensor/1 -> Bus Selector11/1
  MG_sensor/1 -> Bus Selector1/1
  Bus Selector1/1 -> VCU_CNT/4(w_MG_PNT_radps)  "<w_MG_PNT_radps>"
  BT_Hi_PNT_sensor/1 -> Bus Selector2/1
  DCDC_PNT_sensor/1 -> Bus Selector3/1
  CATH_sensor/1 -> Bus Selector4/1
  Bus Selector2/1 -> VCU_CNT/5(SOC_BT_Hi_PNT_per)  "<SOC_BT_Hi_PNT_per>"
  Bus Selector4/1 -> VCU_CNT/6(P_HVAC_PNT_W)  "<P_HVAC_PNT_W>"
  Bus Selector3/1 -> VCU_CNT/7(P_DCDC_PNT_W)  "<P_DCDC_PNT_W>"

== system EV_thermal_charger_2015a_jmaab_Can02/Vehicle/DCDC_PNT/DCDC_PNT ==
  note: 降圧指令
  note: 降圧
  note: DCDC効率計算
  V_BT_Hi_PNT_V : Inport
  V_BT_Lo_PNT_V : Inport  Port=2
  Add : Sum  Inputs=+-
  Constant3 : Constant  Value=DCDC_PNT_eta_conv_lo
  Controller : Subsystem
  Divide : Product  Inputs=/*
  Divide2 : Product  Inputs=/*
  Gain : Gain  Gain=-1
  Gain2 : Gain  Gain=-1
  P_cal : METI_Lib_vehicle_model/P_cal  Type_energy=電気  Type_output_energy=出力  Power_name=Po_  t_Workspace_Name=EL_PNT_DCDC_HI  P_VariableName=Po_EL_PNT_DCDC_HI  Across_VariableName=V_EL_PNT_DCDC_HI  Throgh_VariableName=I_EL_PNT_DCDC_HI
  P_cal5 : METI_Lib_vehicle_model/P_cal  Type_energy=電気  Type_output_energy=損失  Power_name=Pl_  t_Workspace_Name=EL_PNT_DCDC_eta_LOSS  P_VariableName=Pl_EL_PNT_DCDC_eta_LOSS  Across_VariableName=V_EL_PNT_DCDC_eta_LOSS  Throgh_VariableName=I_EL_PNT_DCDC_eta_LOSS
  P_cal6 : METI_Lib_vehicle_model/P_cal  Type_energy=電気  Type_output_energy=損失  Power_name=Pl_  t_Workspace_Name=EL_PNT_DCDC_RESI_LOSS  P_VariableName=Pl_EL_PNT_DCDC_RESI_LOSS  Across_VariableName=V_EL_PNT_DCDC_RESI_LOSS  Throgh_VariableName=I_EL_PNT_DCDC_RESI_LOSS
  P_cal7 : METI_Lib_vehicle_model/P_cal  Type_energy=電気  Type_output_energy=出力  Power_name=Po_  t_Workspace_Name=EL_PNT_DCDC_LO  P_VariableName=Po_EL_PNT_DCDC_LO  Across_VariableName=V_EL_PNT_DCDC_LO  Throgh_VariableName=I_EL_PNT_DCDC_LO
  Product1 : Product  RndMeth=Zero
  Product3 : Product  RndMeth=Zero
  Terminator{1..3,5} (4 alike) : Terminator
  eta_cal1 : METI_Lib_vehicle_model/eta_cal2
  resi1 : Subsystem
  降圧目標1 : Constant  Value=DCDC_PNT_Vtgt_conv_lo
  P_DCDC_PNT_W : Outport
  I_DCDC_PNT_Hi_A : Outport  Port=2
  I_DCDC_PNT_Lo_A : Outport  Port=3
  wires:
  V_BT_Hi_PNT_V/1 -> P_cal/1, Controller/2(V), Product3/2, Divide/1
  Controller/1(Gain) -> Product3/1
  Constant3/1 -> eta_cal1/1
  P_cal7/1 -> Terminator1/1
  P_cal5/1 -> Terminator3/1
  P_cal/1 -> Terminator5/1
  Product3/1 -> Product1/1, Add/1, P_cal5/1, Divide2/1
  Add/1 -> resi1/1(In1), P_cal6/1
  V_BT_Lo_PNT_V/1 -> P_cal7/1, Add/2
  resi1/1(Out1) -> I_DCDC_PNT_Lo_A/1, P_cal7/2, Product1/2, P_cal6/2  "I_DCDC_PNT_Lo_A"
  P_cal6/1 -> Terminator2/1
  降圧目標1/1 -> Controller/1(Target V)
  Product1/1 -> eta_cal1/2
  Divide2/1 -> P_cal5/2
  Divide/1 -> P_cal/2, Gain/1
  Gain2/1 -> Divide2/2
  eta_cal1/1 -> Gain2/1
  Gain/1 -> I_DCDC_PNT_Hi_A/1  "I_DCDC_PNT_Hi_A"
  eta_cal1/2 -> P_DCDC_PNT_W/1, Divide/2

== system EV_thermal_charger_2015a_jmaab_Can02/Vehicle/DTTH/DTTH_PNT ==
  note: DFブロックへ
      | 放熱する熱量
  note: DFからの熱量
  note: モーターハウジングからの熱量
  note: 大気へ
      | 放熱する熱量
  note: 大気へ
      | 放熱する熱量
  note: TMからの熱量
  note: 空調システムからの熱量
  note: ガイドラインでI/Fが定義されているので
      | InOutのI/Fのみ仮設置
  PHI_DF_PNT_W : Inport
  PHI_TM_PNT_W : Inport  Port=2
  "PHI_CATH_PNT_PTTH_W " : Inport  Port=3
  PHI_MGTH_PNT_PTTH_W : Inport  Port=4
  ATM_DTTH : Inport  Port=5
  <ini_T_Environment_Outside_degC> : Inport  Port=6
  <add_T_Environment_PTTH_ELTH_degC> : Inport  Port=7
  Add : Sum
  Bus Selector : BusSelector  OutputSignals=T_ATM_PNT_DF_K,T_ATM_PNT_TM_K
  DFTH_PNT : Subsystem
      mask Display: image(imread('picture\differential.png'))
  Ground : Ground
  K->degC6 : Subsystem
  TMTH_PNT : Subsystem
      mask Display: image(imread('picture\image\transmission02.jpg'))
  Terminator : Terminator
  T_TMTH_PNT_TM_K : Outport
  T_DFTH_PNT_TM_K : Outport  Port=2
  T_TMTH_PNT_ELTH_K : Outport  Port=3
  "PHI_DFTH_PNT_ATM_W " : Outport  Port=4
  "PHI_TMTH_PNT_ATM_W " : Outport  Port=5
  T_TMTH_PNT_TF_degC : Outport  Port=6
  T_PTTH_PNT_CATH_K : Outport  Port=7
  wires:
  TMTH_PNT/5(T_TF_K) -> K->degC6/1(K)
  DFTH_PNT/3("PHI_DFTH_PNT_TMTH_W ") -> TMTH_PNT/5("PHI_DFTH_PNT_TMTH_W ")
  TMTH_PNT/1(T_TMTH_PNT_DFTH_K) -> DFTH_PNT/4("T_TMTH_PNT_DFTH_K ")
  PHI_DF_PNT_W/1 -> DFTH_PNT/3(PHI_DF_PNT_W)
  DFTH_PNT/2(T_DFTH_PNT_TM_K) -> T_DFTH_PNT_TM_K/1
  TMTH_PNT/2(PHI_TMTH_PNT_ATM_W) -> "PHI_TMTH_PNT_ATM_W "/1
  K->degC6/1(degC) -> T_TMTH_PNT_TF_degC/1
  TMTH_PNT/4("T_TMTH_PNT_TM_K ") -> T_TMTH_PNT_TM_K/1
  PHI_TM_PNT_W/1 -> TMTH_PNT/2(PHI_TM_PNT_W)
  TMTH_PNT/3(T_TMTH_PNT_ELTH_K) -> T_TMTH_PNT_ELTH_K/1
  <add_T_Environment_PTTH_ELTH_degC>/1 -> Add/2
  <ini_T_Environment_Outside_degC>/1 -> Add/1
  Add/1 -> DFTH_PNT/1(Temp_ini), TMTH_PNT/1(Temp_ini)
  PHI_MGTH_PNT_PTTH_W/1 -> TMTH_PNT/3("PHI_MGTH_PNT_PTTH_W ")
  Ground/1 -> T_PTTH_PNT_CATH_K/1  "T_PTTH_PNT_CATH_K"
  "PHI_CATH_PNT_PTTH_W "/1 -> Terminator/1
  DFTH_PNT/1("PHI_DFTH_PNT_ATM_W ") -> "PHI_DFTH_PNT_ATM_W "/1
  ATM_DTTH/1 -> Bus Selector/1
  Bus Selector/1 -> DFTH_PNT/2("T_ATM_PNT_DF_K ")  "<T_ATM_PNT_DF_K>"
  Bus Selector/2 -> TMTH_PNT/4("T_ATM_PNT_TM_K ")  "<T_ATM_PNT_TM_K>"

== system EV_thermal_charger_2015a_jmaab_Can02/Vehicle/DT_PNT/DF_PNT ==
  "ｗ_TR_PNT_radps " : Inport
  w_TM_PNT_DN_radps : Inport  Port=2
  "T_DFTH_PNT_TM_K " : Inport  Port=3
  Constant4 : Constant  Value=1 / DF_PNT_DF_gear
  DriveShaft : Subsystem
  Gain : Gain  Gain=-1
  Product4 : Product  Inputs=**  RndMeth=Zero
  Product7 : Product  Inputs=**  RndMeth=Zero
  Q_cal1 : METI_Lib_vehicle_model/P_cal  Type_energy=回転運動  Type_output_energy=出力  Power_name=Po_  t_Workspace_Name=DF_PNT_MECK  P_VariableName=Po_DF_PNT_MECK  Across_VariableName=w_DF_PNT_MECK  Throgh_VariableName=tq_DF_PNT_MECK
  Q_cal4 : METI_Lib_vehicle_model/P_cal  Type_energy=回転運動  Type_output_energy=損失  Power_name=Pl_  t_Workspace_Name=DF_PNT_MECK_LOSS  P_VariableName=Pl_DF_PNT_MECK_LOSS  Across_VariableName=w_DF_PNT_MECK_LOSS  Throgh_VariableName=tq_DF_PNT_MECK_LOSS
  Terminator1 : Terminator
  Terminator3 : Terminator
  eta_DF : Constant  Value=DF_PNT_eta_DF
  eta_cal : METI_Lib_vehicle_model/eta_cal
  Trq_DF_PNT_UP_Nm : Outport
  Trq_DF_PNT_DN_Nm : Outport  Port=2
  "PHI_DF_PNT_W " : Outport  Port=3
  wires:
  w_TM_PNT_DN_radps/1 -> Product4/2, Q_cal4/1, Q_cal1/1
  eta_DF/1 -> eta_cal/1
  eta_cal/2 -> Trq_DF_PNT_UP_Nm/1, Q_cal1/2  "Trq_DF_PNT_UP_Nm"
  eta_cal/1 -> Q_cal4/2
  Q_cal1/1 -> Terminator3/1
  Q_cal4/1 -> Gain/1
  Product7/1 -> eta_cal/2
  Constant4/1 -> Product4/1, Product7/1
  Product4/1 -> DriveShaft/1("w_DF_PNT_radps ")
  DriveShaft/1("Trq_DF_PNT_Nm ") -> Product7/2
  Gain/1 -> "PHI_DF_PNT_W "/1  "PHI_DF_PNT_W"
  "T_DFTH_PNT_TM_K "/1 -> Terminator1/1
  DriveShaft/2(Trq_DF_PNT_DN_Nm) -> Trq_DF_PNT_DN_Nm/1  "Trq_DF_PNT_DN_Nm"
  "ｗ_TR_PNT_radps "/1 -> DriveShaft/2("w_TR_PNT_radps ")

== system EV_thermal_charger_2015a_jmaab_Can02/Vehicle/DT_PNT/TM_PNT ==
  Trq_DF_PNT_UP_Nm : Inport
  "Trq_MG_PNT_Nm " : Inport  Port=2
  T_TMTH_PNT_TM_K : Inport  Port=3
  Constant4 : Constant  Value=TM_PNT_ratio_MG2_gear
  Flywheel1 : Subsystem
  Product4 : Product  Inputs=**  RndMeth=Zero
  Product7 : Product  Inputs=**  RndMeth=Zero
  Q_cal1 : METI_Lib_vehicle_model/P_cal  Type_energy=回転運動  Type_output_energy=出力  Power_name=Po_  t_Workspace_Name=TM_PNT_MECK  P_VariableName=Po_TM_PNT_MECK  Across_VariableName=w_TM_PNT_MECK  Throgh_VariableName=tq_TM_PNT_MECK
  Q_cal4 : METI_Lib_vehicle_model/P_cal  Type_energy=回転運動  Type_output_energy=損失  Power_name=Pl_  t_Workspace_Name=TM_PNT_MECK_LOSS  P_VariableName=Pl_TM_PNT_MECK_LOSS  Across_VariableName=w_TM_PNT_MECK_LOSS  Throgh_VariableName=tq_TM_PNT_MECK_LOSS
  Terminator1 : Terminator
  Terminator2 : Terminator
  eta_DF : Constant  Value=TM_PNT_eta_MG2_gear
  eta_cal_InHi : METI_Lib_vehicle_model/eta_cal_InHi
  "w_TM_PNT_DN_radps " : Outport
  PHI_TM_PNT_W : Outport  Port=2
  w_TM_PNT_UP_radps : Outport  Port=3
  wires:
  Q_cal1/1 -> Terminator1/1
  "Trq_MG_PNT_Nm "/1 -> Q_cal1/2, eta_cal_InHi/2
  Flywheel1/1(w_TM_PNT_DN_radps) -> "w_TM_PNT_DN_radps "/1  "w_TM_PNT_DN_radps"
  Trq_DF_PNT_UP_Nm/1 -> Flywheel1/1(Trq_DF_PNT_UP_Nm)
  eta_DF/1 -> eta_cal_InHi/1
  eta_cal_InHi/1 -> Q_cal4/2
  Constant4/1 -> Product7/1, Product4/1
  eta_cal_InHi/2 -> Product7/2
  Product4/1 -> Q_cal1/1, Q_cal4/1, w_TM_PNT_UP_radps/1  "w_TM_PNT_UP_radps"
  Flywheel1/2("w_ROT_TM_Flywheel_UP ") -> Product4/2
  Product7/1 -> Flywheel1/2(Trq_TM_Flywheel_UP)
  Q_cal4/1 -> PHI_TM_PNT_W/1  "PHI_TM_PNT_W"
  T_TMTH_PNT_TM_K/1 -> Terminator2/1

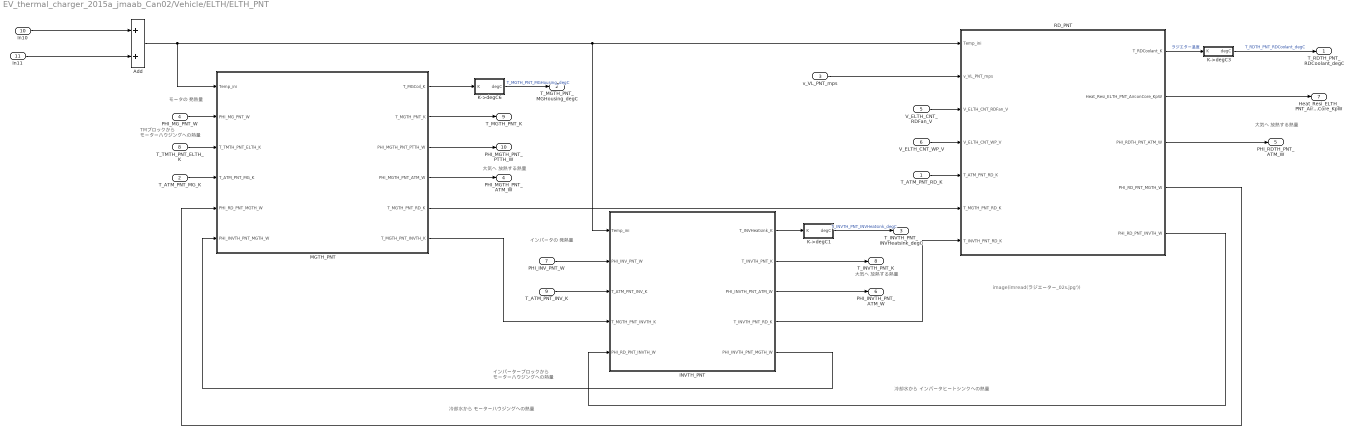
== system EV_thermal_charger_2015a_jmaab_Can02/Vehicle/ELTH/ELTH_PNT ==
  note: image(imread('ラジエーター_02s.jpg'))
  note: 大気へ
      | 放熱する熱量
  note: 冷却水から
      | モーターハウジングへの熱量
  note: インバーターブロックから
      | モーターハウジングへの熱量
  note: 大気へ
      | 放熱する熱量
  note: 冷却水から
      | インバータヒートシンクへの熱量
  note: モータの
      | 発熱量
  note: TMブロックから
      | モーターハウジングへの熱量
  note: インバータの
      | 発熱量
  note: 大気へ
      | 放熱する熱量
  T_ATM_PNT_RD_K : Inport
  T_ATM_PNT_MG_K : Inport  Port=2
  v_VL_PNT_mps : Inport  Port=3
  PHI_MG_PNT_W : Inport  Port=4
  V_ELTH_CNT_RDFan_V : Inport  Port=5
  V_ELTH_CNT_WP_V : Inport  Port=6
  PHI_INV_PNT_W : Inport  Port=7
  T_TMTH_PNT_ELTH_K : Inport  Port=8
  T_ATM_PNT_INV_K : Inport  Port=9
  In10 : Inport  Port=10
  In11 : Inport  Port=11
  Add : Sum
  INVTH_PNT : Subsystem
      mask Display: image(imread('inverter02s.jpg'))
  K->degC1 : Subsystem
  K->degC3 : Subsystem
  K->degC6 : Subsystem
  MGTH_PNT : Subsystem
      mask Display: image(imread('motor_drive_system03.png'))
  RD_PNT : Subsystem
  T_RDTH_PNT_RDCoolant_degC : Outport
  T_MGTH_PNT_MGHousing_degC : Outport  Port=2
  T_INVTH_PNT_INVHeatsink_degC : Outport  Port=3
  "PHI_MGTH_PNT_ATM_W " : Outport  Port=4
  "PHI_RDTH_PNT_ATM_W " : Outport  Port=5
  "PHI_INVTH_PNT_ATM_W " : Outport  Port=6
  Heat_Resi_ELTH_PNT_AirconCore_KpW : Outport  Port=7
  T_INVTH_PNT_K : Outport  Port=8
  T_MGTH_PNT_K : Outport  Port=9
  PHI_MGTH_PNT_PTTH_W : Outport  Port=10
  wires:
  v_VL_PNT_mps/1 -> RD_PNT/2(v_VL_PNT_mps)
  V_ELTH_CNT_RDFan_V/1 -> RD_PNT/3(V_ELTH_CNT_RDFan_V)
  RD_PNT/1(T_RDCoolant_K) -> K->degC3/1(K)  "ラジエター温度"
  MGTH_PNT/1(T_MGCoil_K) -> K->degC6/1(K)
  PHI_MG_PNT_W/1 -> MGTH_PNT/2(PHI_MG_PNT_W)
  MGTH_PNT/2(T_MGTH_PNT_K) -> T_MGTH_PNT_K/1
  T_TMTH_PNT_ELTH_K/1 -> MGTH_PNT/3(T_TMTH_PNT_ELTH_K)
  MGTH_PNT/3(PHI_MGTH_PNT_PTTH_W) -> PHI_MGTH_PNT_PTTH_W/1
  MGTH_PNT/6(T_MGTH_PNT_INVTH_K) -> INVTH_PNT/4(T_MGTH_PNT_INVTH_K)
  INVTH_PNT/5(PHI_INVTH_PNT_MGTH_W) -> MGTH_PNT/6(PHI_INVTH_PNT_MGTH_W)
  INVTH_PNT/2(T_INVTH_PNT_K) -> T_INVTH_PNT_K/1
  PHI_INV_PNT_W/1 -> INVTH_PNT/2(PHI_INV_PNT_W)
  INVTH_PNT/4(T_INVTH_PNT_RD_K) -> RD_PNT/7(T_INVTH_PNT_RD_K)
  RD_PNT/5(PHI_RD_PNT_INVTH_W) -> INVTH_PNT/5(PHI_RD_PNT_INVTH_W)
  MGTH_PNT/5(T_MGTH_PNT_RD_K) -> RD_PNT/6(T_MGTH_PNT_RD_K)
  RD_PNT/4(PHI_RD_PNT_MGTH_W) -> MGTH_PNT/5(" PHI_RD_PNT_MGTH_W")
  T_ATM_PNT_INV_K/1 -> INVTH_PNT/3(T_ATM_PNT_INV_K)
  INVTH_PNT/3(PHI_INVTH_PNT_ATM_W) -> "PHI_INVTH_PNT_ATM_W "/1
  T_ATM_PNT_RD_K/1 -> RD_PNT/5(T_ATM_PNT_RD_K)
  RD_PNT/3(PHI_RDTH_PNT_ATM_W) -> "PHI_RDTH_PNT_ATM_W "/1
  T_ATM_PNT_MG_K/1 -> MGTH_PNT/4(T_ATM_PNT_MG_K)
  MGTH_PNT/4(PHI_MGTH_PNT_ATM_W) -> "PHI_MGTH_PNT_ATM_W "/1
  INVTH_PNT/1(T_INVHeatsink_K) -> K->degC1/1(K)
  V_ELTH_CNT_WP_V/1 -> RD_PNT/4(V_ELTH_CNT_WP_V)
  K->degC3/1(degC) -> T_RDTH_PNT_RDCoolant_degC/1  "T_RDTH_PNT_RDCoolant_degC"
  In11/1 -> Add/2
  Add/1 -> MGTH_PNT/1(Temp_ini), INVTH_PNT/1(Temp_ini), RD_PNT/1(Temp_ini)
  K->degC6/1(degC) -> T_MGTH_PNT_MGHousing_degC/1  "T_MGTH_PNT_MGHousing_degC"
  K->degC1/1(degC) -> T_INVTH_PNT_INVHeatsink_degC/1  "T_INVTH_PNT_INVHeatsink_degC"
  RD_PNT/2(Heat_Resi_ELTH_PNT_AirconCore_KpW) -> Heat_Resi_ELTH_PNT_AirconCore_KpW/1
  In10/1 -> Add/1

== system EV_thermal_charger_2015a_jmaab_Can02/Vehicle/EL_PNT/Divide_0wari1 ==
  In1 : Inport
  In2 : Inport  Port=2
  Constant : Constant  Value=0
  Constant1 : Constant
  Constant2 : Constant  Value=0
  Divide : Product  Inputs=*/
  Logical Operator : Logic  Operator=OR  AllPortsSameDT=off  OutDataTypeStr=boolean
  Relational Operator : RelationalOperator  Operator=>  OutDataTypeStr=boolean
  Relational Operator1 : RelationalOperator  Operator=<  OutDataTypeStr=boolean
  Switch : Switch  Criteria=u2 > Threshold  Threshold=0.5
  Switch1 : Switch  Criteria=u2 > Threshold  Threshold=0.5
  Out1 : Outport
  wires:
  In1/1 -> Divide/1
  Divide/1 -> Switch1/1
  In2/1 -> Relational Operator1/1, Relational Operator/1, Switch/1
  Constant/1 -> Relational Operator1/2, Relational Operator/2
  Relational Operator/1 -> Logical Operator/1
  Relational Operator1/1 -> Logical Operator/2
  Switch/1 -> Divide/2
  Logical Operator/1 -> Switch1/2, Switch/2
  Constant1/1 -> Switch/3
  Constant2/1 -> Switch1/3
  Switch1/1 -> Out1/1

== system EV_thermal_charger_2015a_jmaab_Can02/Vehicle/EL_PNT/Lo_body_elec_load_resi ==

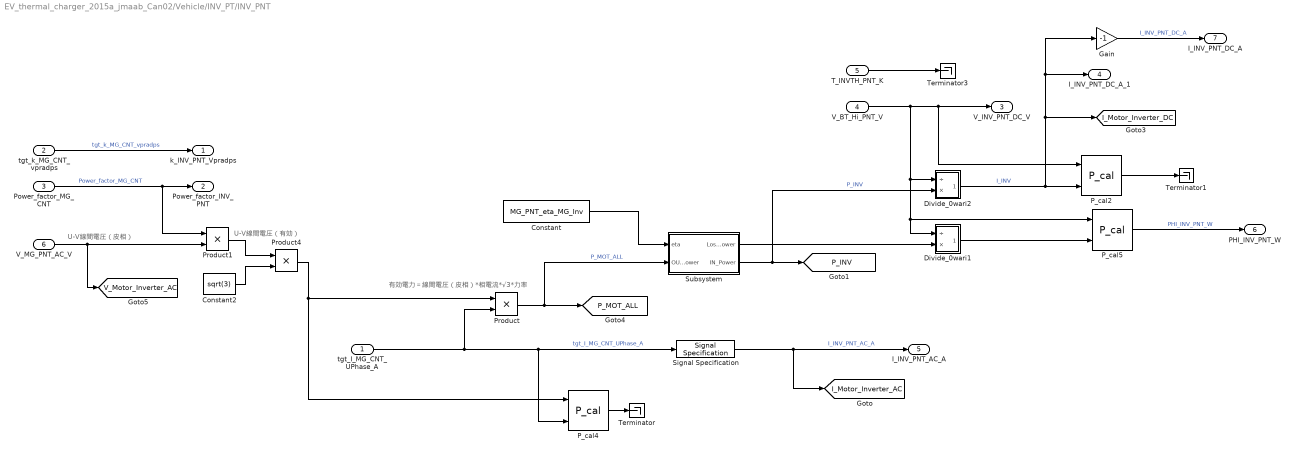
== system EV_thermal_charger_2015a_jmaab_Can02/Vehicle/INV_PT/INV_PNT ==
  note: U-V線間電圧（皮相）
  note: 有効電力＝線間電圧（皮相）*相電流*√3*力率
  note: U-V線間電圧（有効）
  tgt_I_MG_CNT_UPhase_A : Inport
  tgt_k_MG_CNT_vpradps : Inport  Port=2
  Power_factor_MG_CNT : Inport  Port=3
  V_BT_Hi_PNT_V : Inport  Port=4
  T_INVTH_PNT_K : Inport  Port=5
  V_MG_PNT_AC_V : Inport  Port=6
  Constant : Constant  Value=MG_PNT_eta_MG_Inv
  Constant2 : Constant  Value=sqrt(3)
  Divide_0wari1 : Subsystem
  Divide_0wari2 : Subsystem
  Gain : Gain  Gain=-1
  P_cal2 : METI_Lib_vehicle_model/P_cal  Type_energy=電気  Type_output_energy=出力  Power_name=Po_  t_Workspace_Name=MG_INV_PNT_DC_ELEC  P_VariableName=Po_MG_INV_PNT_DC_ELEC  Across_VariableName=V_MG_INV_PNT_DC_ELEC  Throgh_VariableName=I_MG_INV_PNT_DC_ELEC
  P_cal4 : METI_Lib_vehicle_model/P_cal  Type_energy=電気  Type_output_energy=出力  Power_name=Po_  t_Workspace_Name=MG_INV_PNT_AC_ELEC  P_VariableName=Po_MG_INV_PNT_AC_ELEC  Across_VariableName=V_MG_INV_PNT_AC_ELEC  Throgh_VariableName=I_MG_INV_PNT_AC_ELEC
  P_cal5 : METI_Lib_vehicle_model/P_cal  Type_energy=電気  Type_output_energy=損失  Power_name=Pl_  t_Workspace_Name=MG_INV_PNT_ELEC_LOSS  P_VariableName=Pl_MG_INV_PNT_ELEC_LOSS  Across_VariableName=V_MG_INV_PNT_ELEC_LOSS  Throgh_VariableName=I_MG_INV_PNT_ELEC_LOSS
  Product : Product
  Product1 : Product
  Product4 : Product
  Signal Specification : SignalSpecification
  Subsystem : Subsystem
  Terminator : Terminator
  Terminator1 : Terminator
  Terminator3 : Terminator
  k_INV_PNT_Vpradps : Outport
  Power_factor_INV_PNT : Outport  Port=2
  V_INV_PNT_DC_V : Outport  Port=3
  I_INV_PNT_DC_A_1 : Outport  Port=4
  I_INV_PNT_AC_A : Outport  Port=5
  PHI_INV_PNT_W : Outport  Port=6
  I_INV_PNT_DC_A : Outport  Port=7
  tag scope: I_Motor_Inverter_AC=global, I_Motor_Inverter_DC=global, P_INV=global, P_MOT_ALL=global, V_Motor_Inverter_AC=global
  wires:
  Constant/1 -> Subsystem/1(eta)
  Subsystem/2(IN_Power) -> [P_INV], Divide_0wari2/2(×)  "P_INV"
  Divide_0wari1/1("　") -> P_cal5/2
  P_cal5/1 -> PHI_INV_PNT_W/1  "PHI_INV_PNT_W"
  Subsystem/1(Loss_Power) -> Divide_0wari1/2(×)
  P_cal4/1 -> Terminator/1
  V_BT_Hi_PNT_V/1 -> P_cal2/1, V_INV_PNT_DC_V/1, Divide_0wari2/1(÷), Divide_0wari1/1(÷), P_cal5/1
  Divide_0wari2/1("　") -> [I_Motor_Inverter_DC], Gain/1, I_INV_PNT_DC_A_1/1, P_cal2/2  "I_INV"
  P_cal2/1 -> Terminator1/1
  Gain/1 -> I_INV_PNT_DC_A/1  "I_INV_PNT_DC_A"
  Product/1 -> [P_MOT_ALL], Subsystem/2(OUT_Power)  "P_MOT_ALL"
  tgt_k_MG_CNT_vpradps/1 -> k_INV_PNT_Vpradps/1  "tgt_k_MG_CNT_vpradps"
  tgt_I_MG_CNT_UPhase_A/1 -> Signal Specification/1, P_cal4/2, Product/2  "tgt_I_MG_CNT_UPhase_A"
  Product4/1 -> Product/1, P_cal4/1
  Power_factor_MG_CNT/1 -> Product1/1, Power_factor_INV_PNT/1  "Power_factor_MG_CNT"
  V_MG_PNT_AC_V/1 -> [V_Motor_Inverter_AC], Product1/2
  T_INVTH_PNT_K/1 -> Terminator3/1
  Constant2/1 -> Product4/2
  Product1/1 -> Product4/1
  Signal Specification/1 -> [I_Motor_Inverter_AC], I_INV_PNT_AC_A/1  "I_INV_PNT_AC_A"
